simulink model "rfkjrtest"  (R2024a)
settings: Solver=VariableStepAuto  StartTime=0.0  StopTime=150  RelTol=1e-3
settings Model: Creator=harounf  LastModifiedBy=JeffZ

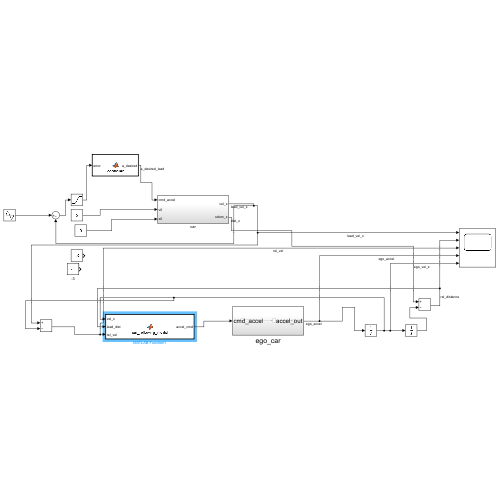
[thumbnail: Simulink's stored preview of the top-level diagram]
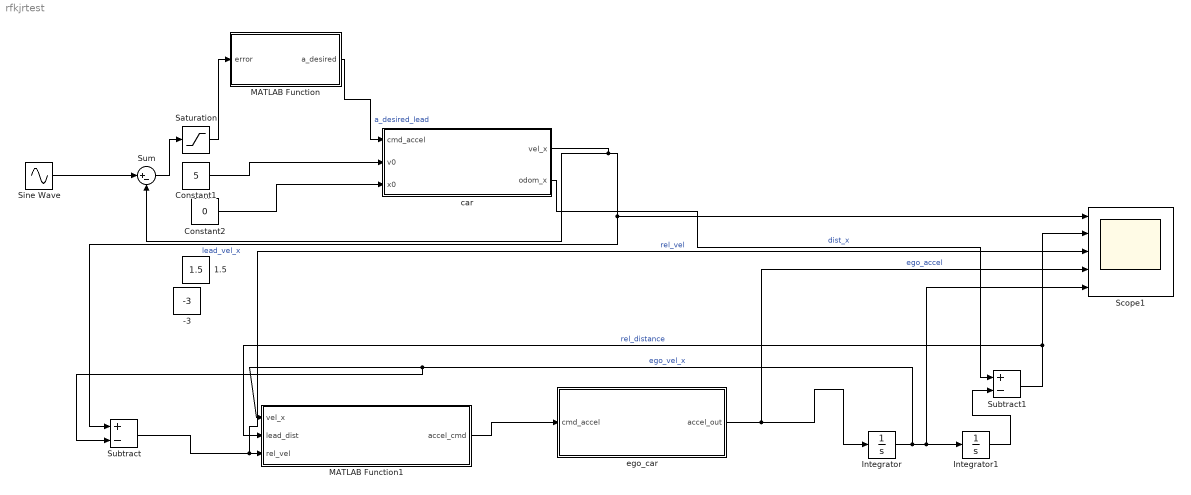
== system rfkjrtest ==
  -3 : Constant  Value=-3
  1.5 : Constant  Value=1.5
  Constant1 : Constant  Value=5
  Constant2 : Constant  Value=0
  Integrator : Integrator
  Integrator1 : Integrator
  MATLAB Function : MATLAB Function  TreatAsAtomicUnit=on
  MATLAB Function1 : MATLAB Function  TreatAsAtomicUnit=on
  Saturation : Saturate  UpperLimit=1.5  LowerLimit=-3
  Scope1 : Scope  NumInputPorts=5
  Sine Wave : Sin  Amplitude=10  Bias=20  Frequency=.25  SampleTime=0
  Subtract : Sum  Inputs=+-
  Subtract1 : Sum  Inputs=+-
  Sum : Sum  Inputs=|+-
  car : Subsystem
  ego_car : Subsystem
  wires:
  MATLAB Function1/1(accel_cmd) -> ego_car/1(cmd_accel)
  ego_car/1(accel_out) -> Scope1/4, Integrator/1  "ego_accel"
  Constant2/1 -> car/3(x0)
  car/1(vel_x) -> Sum/2, Subtract/1, Scope1/1  "lead_vel_x"
  Constant1/1 -> car/2(v0)
  Sum/1 -> Saturation/1
  car/2(odom_x) -> Subtract1/1  "dist_x"
  Integrator/1 -> Scope1/5, Integrator1/1, Subtract/2, MATLAB Function1/1(vel_x)  "ego_vel_x"
  Subtract/1 -> Scope1/3, MATLAB Function1/3(rel_vel)  "rel_vel"
  Integrator1/1 -> Subtract1/2
  Subtract1/1 -> Scope1/2, MATLAB Function1/2(lead_dist)  "rel_distance"
  Saturation/1 -> MATLAB Function/1(error)
  MATLAB Function/1(a_desired) -> car/1(cmd_accel)  "a_desired_lead"
  Sine Wave/1 -> Sum/1

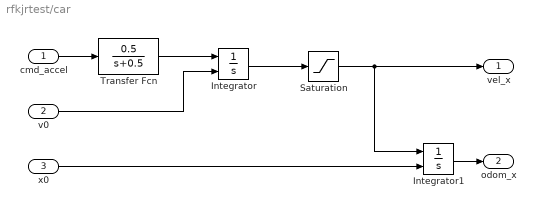
== system rfkjrtest/car ==
  cmd_accel : Inport
  v0 : Inport  Port=2
  x0 : Inport  Port=3
  Integrator : Integrator  InitialConditionSource=external
  Integrator1 : Integrator  InitialConditionSource=external
  Saturation : Saturate  UpperLimit=80  LowerLimit=0
  Transfer Fcn : TransferFcn  Numerator=[0.5]  Denominator=[1 0.5]
  vel_x : Outport
  odom_x : Outport  Port=2
  wires:
  v0/1 -> Integrator/2
  cmd_accel/1 -> Transfer Fcn/1
  Transfer Fcn/1 -> Integrator/1
  Integrator1/1 -> odom_x/1
  Integrator/1 -> Saturation/1
  x0/1 -> Integrator1/2
  Saturation/1 -> vel_x/1, Integrator1/1

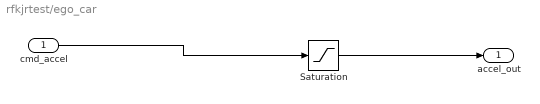
== system rfkjrtest/ego_car ==
  cmd_accel : Inport
  Saturation : Saturate  UpperLimit=5  LowerLimit=-5
  accel_out : Outport
  wires:
  Saturation/1 -> accel_out/1
  cmd_accel/1 -> Saturation/1

== matlab function rfkjrtest/MATLAB Function1 ==
  data: accel_cmd output; vel_x input; lead_dist input; rel_vel input
function accel_cmd = car_following_model(vel_x, lead_dist, rel_vel)
    % Eco-Driving Car Following Model with Extended Logic for Large Lead Distance
    % Inputs:
    %   vel_x: Velocity of the ego vehicle (m/s)
    %   lead_dist: Distance to the lead vehicle (m)
    %   rel_vel: Relative velocity between the ego and lead vehicle (lead_vel - ego_vel) (m/s)
    %
    % Output:
    %   accel_cmd: Desired acceleration for the ego vehicle (m/s^2)

    % Parameters for maintaining a safe following distance
    alpha = .5;        % Proportional gain for distance maintenance
    tau = 2.5;          % Desired time gap (seconds)
    
    % Parameters for smooth driving
    beta_acc = 0.05;     % Proportional gain for acceleration smoothness
    beta_dec = 0.25;     % Proportional gain for deceleration smoothness
    max_acc = 1.5;      % Maximum acceleration allowed (m/s^2)
    max_dec = -2.0;     % Maximum deceleration allowed (m/s^2)
    
    % Constant speed parameters
    eco_speed = 20;     % Eco-friendly cruising speed (m/s)
    max_lead_dist = 100; % Maximum distance before ego maintains constant speed (meters)

    % Calculate the desired safe distance using the time gap policy
    desired_space_gap = vel_x * tau;

    % Calculate the error in the current space gap
    gap_error = lead_dist - desired_space_gap;

    % Basic constant time gap control law for maintaining safe distance
    accel_gap_control = alpha * gap_error;

    % Smooth adjustment to avoid abrupt acceleration and braking
    if rel_vel > 0
        % Ego vehicle should accelerate to close the gap
        accel_smooth_control = beta_acc * rel_vel;
    else
        % Ego vehicle should decelerate to maintain gap smoothly
        accel_smooth_control = beta_dec * rel_vel;
    end

    % Desired acceleration is a combination of gap maintenance and smoothness control
    accel_cmd = accel_gap_control + accel_smooth_control;

    % Additional logic for when the lead car is too far away
    if lead_dist > max_lead_dist
        % Maintain a constant speed at the eco-friendly rate
        if vel_x < eco_speed
            % Accelerate to reach eco speed
            accel_cmd = beta_acc * (eco_speed - vel_x);
        elseif vel_x > eco_speed
            % Decelerate to reach eco speed
            accel_cmd = beta_dec * (eco_speed - vel_x);
        else
            % No change in acceleration needed if at desired eco speed
            accel_cmd = 0;
        end
    end

    % Limit acceleration to ensure eco-friendly driving behavior
    accel_cmd = min(max(accel_cmd, max_dec), max_acc);
end

== matlab function rfkjrtest/MATLAB Function ==
  data: error input; a_desired output
function a_desired = controller(error)

a_desired = .3*error;
